simulink model "rippleCarryAdder"  (R2015a)
settings: Solver=ode1  StartTime=0.0  StopTime=10.0  FixedStep=1  RelTol=1e-3
libraries: commutil2 x3
settings Model: Creator=Osmaz  LastModifiedBy=Osmaz

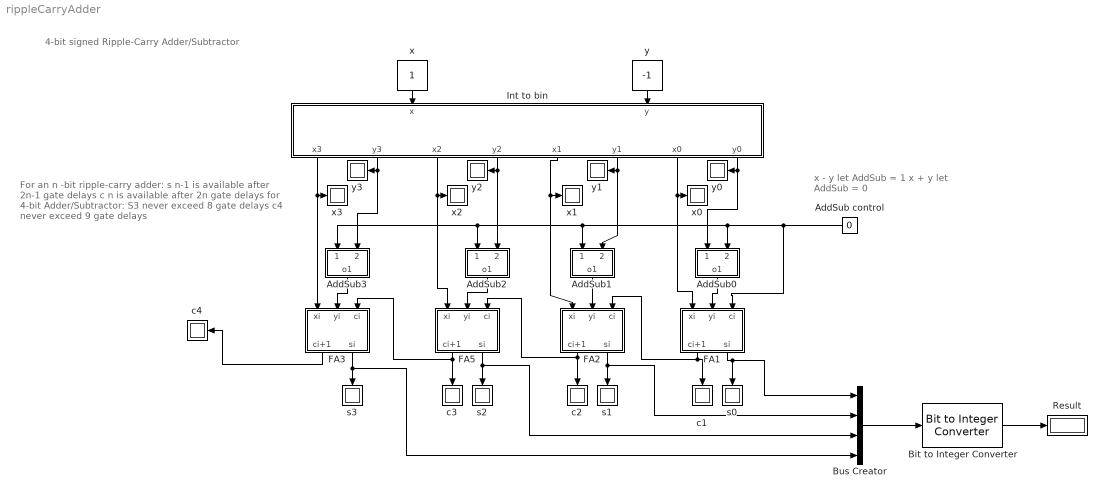
== system rippleCarryAdder ==
  note: For an n -bit ripple-carry adder:
      | s n-1 is available after 2n-1 gate delays
      | c n is available after 2n gate delays
      |
      | for 4-bit Adder/Subtractor:
      | S3 never exceed 8 gate delays
      | c4 never exceed 9 gate delays
  note: 4-bit signed Ripple-Carry Adder/Subtractor
  note: x - y let AddSub = 1
      | x + y let AddSub = 0
  AddSub control : Constant  Value=0  OutMin=0  OutMax=1  OutDataTypeStr=boolean
  AddSub0 : Subsystem
  AddSub1 : Subsystem
  AddSub2 : Subsystem
  AddSub3 : Subsystem
  Bit to Integer Converter : commutil2/Bit to Integer Converter  nbits=4  bitOrder=LSB first  signedOutputValues=Signed  outDtype=Inherit via internal rule  outDtypeSigned=Inherit via internal rule
  Bus Creator : BusCreator  DialogController=Simulink.DDGSource_BusCreator
  FA1 : Subsystem
  FA2 : Subsystem
  FA3 : Subsystem
  FA5 : Subsystem
  Int to bin : Subsystem
  Result : Display
  c{1..4} (4 alike) : Display
  s{0..3} (4 alike) : Display
  x : Constant  OutMin=-8  OutMax=7  OutDataTypeStr=int8  SampleTime=1
  x{0..3} (4 alike) : Display
  y : Constant  Value=-1  OutMin=-8  OutMax=7  OutDataTypeStr=int8  SampleTime=1
  y{0..3} (4 alike) : Display
  wires:
  Int to bin/7(x0) -> x0/1, FA1/1(xi)
  AddSub control/1 -> FA1/3(ci), AddSub1/1(1), AddSub3/1(1), AddSub2/1(1), AddSub0/2(2)
  FA1/2(si) -> s0/1, Bus Creator/1
  Int to bin/5(x1) -> FA2/1(xi), x1/1
  FA2/2(si) -> Bus Creator/2, s1/1
  FA1/1(ci+1) -> c1/1, FA2/3(ci)
  Int to bin/3(x2) -> FA5/1(xi), x2/1
  FA5/2(si) -> s2/1, Bus Creator/3
  FA2/1(ci+1) -> FA5/3(ci), c2/1
  Int to bin/1(x3) -> x3/1, FA3/1(xi)
  FA3/2(si) -> s3/1, Bus Creator/4
  FA5/1(ci+1) -> FA3/3(ci), c3/1
  FA3/1(ci+1) -> c4/1
  Bit to Integer Converter/1 -> Result/1
  Bus Creator/1 -> Bit to Integer Converter/1
  x/1 -> Int to bin/1(x)
  y/1 -> Int to bin/2(y)
  Int to bin/8(y0) -> AddSub0/1(1), y0/1
  Int to bin/6(y1) -> AddSub1/2(2), y1/1
  Int to bin/4(y2) -> y2/1, AddSub2/2(2)
  Int to bin/2(y3) -> AddSub3/2(2), y3/1
  AddSub1/1(o1) -> FA2/2(yi)
  AddSub2/1(o1) -> FA5/2(yi)
  AddSub3/1(o1) -> FA3/2(yi)
  AddSub0/1(o1) -> FA1/2(yi)

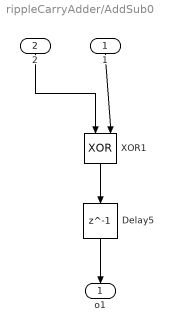
== system rippleCarryAdder/AddSub0 ==
  1 : Inport
  2 : Inport  Port=2
  Delay5 : Delay  DialogController=Simulink.DDGSource  DelayLength=1  InitialCondition=0  InputProcessing=Inherited
  XOR1 : Logic  Operator=XOR  IconShape=distinctive  AllPortsSameDT=off  OutDataTypeStr=boolean
  o1 : Outport
  wires:
  1/1 -> XOR1/2
  2/1 -> XOR1/1
  XOR1/1 -> Delay5/1
  Delay5/1 -> o1/1

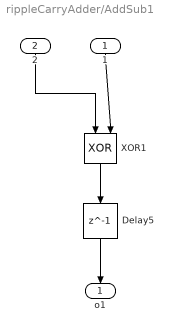
== system rippleCarryAdder/AddSub1 ==
  1 : Inport
  2 : Inport  Port=2
  Delay5 : Delay  DelayLength=1  InitialCondition=0  InputProcessing=Inherited
  XOR1 : Logic  Operator=XOR  IconShape=distinctive  AllPortsSameDT=off  OutDataTypeStr=boolean
  o1 : Outport
  wires:
  1/1 -> XOR1/2
  2/1 -> XOR1/1
  XOR1/1 -> Delay5/1
  Delay5/1 -> o1/1

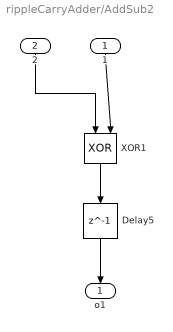
== system rippleCarryAdder/AddSub2 ==
  1 : Inport
  2 : Inport  Port=2
  Delay5 : Delay  DelayLength=1  InitialCondition=0  InputProcessing=Inherited
  XOR1 : Logic  Operator=XOR  IconShape=distinctive  AllPortsSameDT=off  OutDataTypeStr=boolean
  o1 : Outport
  wires:
  1/1 -> XOR1/2
  2/1 -> XOR1/1
  XOR1/1 -> Delay5/1
  Delay5/1 -> o1/1

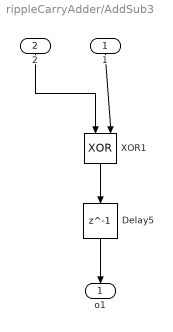
== system rippleCarryAdder/AddSub3 ==
  1 : Inport
  2 : Inport  Port=2
  Delay5 : Delay  DelayLength=1  InitialCondition=0  InputProcessing=Inherited
  XOR1 : Logic  Operator=XOR  IconShape=distinctive  AllPortsSameDT=off  OutDataTypeStr=boolean
  o1 : Outport
  wires:
  1/1 -> XOR1/2
  2/1 -> XOR1/1
  XOR1/1 -> Delay5/1
  Delay5/1 -> o1/1

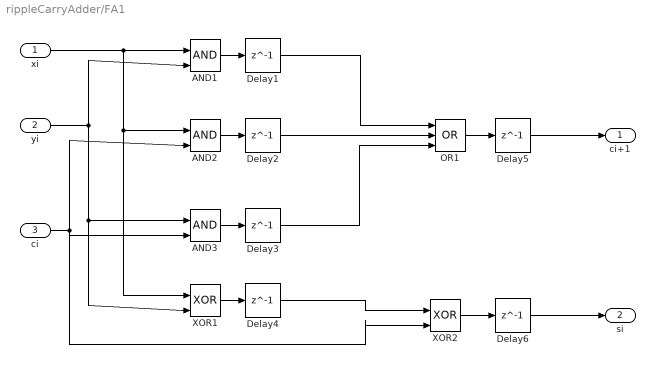
== system rippleCarryAdder/FA1 ==
  xi : Inport
  yi : Inport  Port=2
  ci : Inport  Port=3
  AND1 : Logic  IconShape=distinctive  AllPortsSameDT=off  OutDataTypeStr=boolean
  AND2 : Logic  IconShape=distinctive  AllPortsSameDT=off  OutDataTypeStr=boolean
  AND3 : Logic  IconShape=distinctive  AllPortsSameDT=off  OutDataTypeStr=boolean
  Delay{1..6} (6 alike) : Delay  DelayLength=1  InitialCondition=0  InputProcessing=Inherited
  OR1 : Logic  Operator=OR  Inputs=3  IconShape=distinctive  AllPortsSameDT=off  OutDataTypeStr=boolean
  XOR1 : Logic  Operator=XOR  IconShape=distinctive  AllPortsSameDT=off  OutDataTypeStr=boolean
  XOR2 : Logic  Operator=XOR  IconShape=distinctive  AllPortsSameDT=off  OutDataTypeStr=boolean
  ci+1 : Outport
  si : Outport  Port=2
  wires:
  Delay1/1 -> OR1/1
  AND1/1 -> Delay1/1
  yi/1 -> AND1/2, XOR1/2, AND3/1
  xi/1 -> AND1/1, XOR1/1, AND2/1
  AND2/1 -> Delay2/1
  Delay2/1 -> OR1/2
  AND3/1 -> Delay3/1
  Delay3/1 -> OR1/3
  ci/1 -> XOR2/2, AND2/2, AND3/2
  OR1/1 -> Delay5/1
  Delay5/1 -> ci+1/1
  Delay6/1 -> si/1
  XOR1/1 -> Delay4/1
  Delay4/1 -> XOR2/1
  XOR2/1 -> Delay6/1

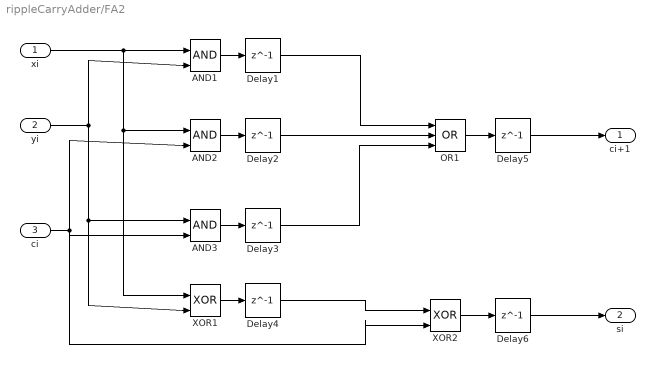
== system rippleCarryAdder/FA2 ==
  xi : Inport
  yi : Inport  Port=2
  ci : Inport  Port=3
  AND1 : Logic  IconShape=distinctive  AllPortsSameDT=off  OutDataTypeStr=boolean
  AND2 : Logic  IconShape=distinctive  AllPortsSameDT=off  OutDataTypeStr=boolean
  AND3 : Logic  IconShape=distinctive  AllPortsSameDT=off  OutDataTypeStr=boolean
  Delay{1..6} (6 alike) : Delay  DelayLength=1  InitialCondition=0  InputProcessing=Inherited
  OR1 : Logic  Operator=OR  Inputs=3  IconShape=distinctive  AllPortsSameDT=off  OutDataTypeStr=boolean
  XOR1 : Logic  Operator=XOR  IconShape=distinctive  AllPortsSameDT=off  OutDataTypeStr=boolean
  XOR2 : Logic  Operator=XOR  IconShape=distinctive  AllPortsSameDT=off  OutDataTypeStr=boolean
  ci+1 : Outport
  si : Outport  Port=2
  wires:
  Delay1/1 -> OR1/1
  AND1/1 -> Delay1/1
  yi/1 -> AND1/2, XOR1/2, AND3/1
  xi/1 -> AND1/1, XOR1/1, AND2/1
  AND2/1 -> Delay2/1
  Delay2/1 -> OR1/2
  AND3/1 -> Delay3/1
  Delay3/1 -> OR1/3
  ci/1 -> XOR2/2, AND2/2, AND3/2
  OR1/1 -> Delay5/1
  Delay5/1 -> ci+1/1
  Delay6/1 -> si/1
  XOR1/1 -> Delay4/1
  Delay4/1 -> XOR2/1
  XOR2/1 -> Delay6/1

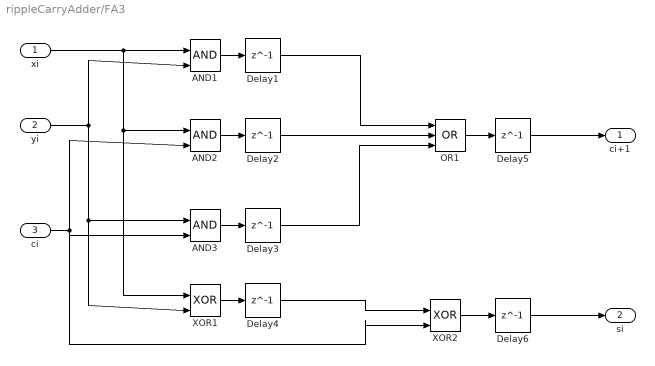
== system rippleCarryAdder/FA3 ==
  xi : Inport
  yi : Inport  Port=2
  ci : Inport  Port=3
  AND1 : Logic  IconShape=distinctive  AllPortsSameDT=off  OutDataTypeStr=boolean
  AND2 : Logic  IconShape=distinctive  AllPortsSameDT=off  OutDataTypeStr=boolean
  AND3 : Logic  IconShape=distinctive  AllPortsSameDT=off  OutDataTypeStr=boolean
  Delay{1..6} (6 alike) : Delay  DelayLength=1  InitialCondition=0  InputProcessing=Inherited
  OR1 : Logic  Operator=OR  Inputs=3  IconShape=distinctive  AllPortsSameDT=off  OutDataTypeStr=boolean
  XOR1 : Logic  Operator=XOR  IconShape=distinctive  AllPortsSameDT=off  OutDataTypeStr=boolean
  XOR2 : Logic  Operator=XOR  IconShape=distinctive  AllPortsSameDT=off  OutDataTypeStr=boolean
  ci+1 : Outport
  si : Outport  Port=2
  wires:
  Delay1/1 -> OR1/1
  AND1/1 -> Delay1/1
  yi/1 -> AND1/2, XOR1/2, AND3/1
  xi/1 -> AND1/1, XOR1/1, AND2/1
  AND2/1 -> Delay2/1
  Delay2/1 -> OR1/2
  AND3/1 -> Delay3/1
  Delay3/1 -> OR1/3
  ci/1 -> XOR2/2, AND2/2, AND3/2
  OR1/1 -> Delay5/1
  Delay5/1 -> ci+1/1
  Delay6/1 -> si/1
  XOR1/1 -> Delay4/1
  Delay4/1 -> XOR2/1
  XOR2/1 -> Delay6/1

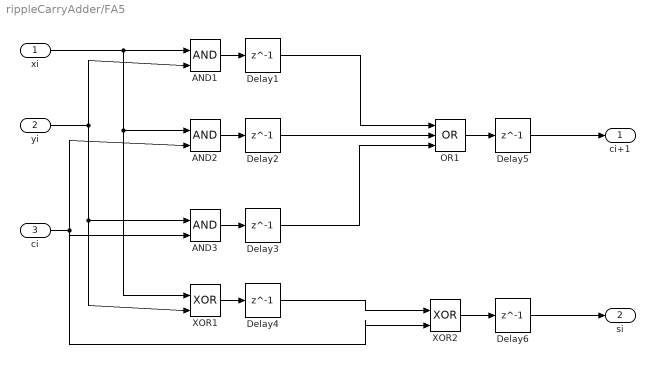
== system rippleCarryAdder/FA5 ==
  xi : Inport
  yi : Inport  Port=2
  ci : Inport  Port=3
  AND1 : Logic  IconShape=distinctive  AllPortsSameDT=off  OutDataTypeStr=boolean
  AND2 : Logic  IconShape=distinctive  AllPortsSameDT=off  OutDataTypeStr=boolean
  AND3 : Logic  IconShape=distinctive  AllPortsSameDT=off  OutDataTypeStr=boolean
  Delay{1..6} (6 alike) : Delay  DelayLength=1  InitialCondition=0  InputProcessing=Inherited
  OR1 : Logic  Operator=OR  Inputs=3  IconShape=distinctive  AllPortsSameDT=off  OutDataTypeStr=boolean
  XOR1 : Logic  Operator=XOR  IconShape=distinctive  AllPortsSameDT=off  OutDataTypeStr=boolean
  XOR2 : Logic  Operator=XOR  IconShape=distinctive  AllPortsSameDT=off  OutDataTypeStr=boolean
  ci+1 : Outport
  si : Outport  Port=2
  wires:
  Delay1/1 -> OR1/1
  AND1/1 -> Delay1/1
  yi/1 -> AND1/2, XOR1/2, AND3/1
  xi/1 -> AND1/1, XOR1/1, AND2/1
  AND2/1 -> Delay2/1
  Delay2/1 -> OR1/2
  AND3/1 -> Delay3/1
  Delay3/1 -> OR1/3
  ci/1 -> XOR2/2, AND2/2, AND3/2
  OR1/1 -> Delay5/1
  Delay5/1 -> ci+1/1
  Delay6/1 -> si/1
  XOR1/1 -> Delay4/1
  Delay4/1 -> XOR2/1
  XOR2/1 -> Delay6/1

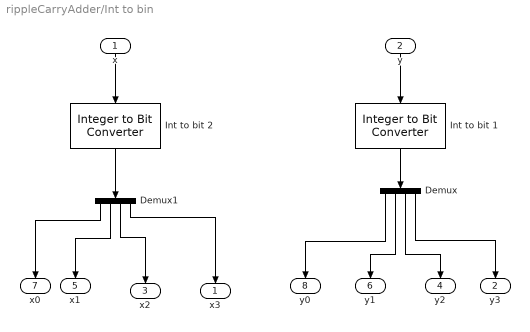
== system rippleCarryAdder/Int to bin ==
  x : Inport
  y : Inport  Port=2
  Demux : Demux
  Demux1 : Demux
  Int to bit 1 : commutil2/Integer to Bit Converter  nbits=4  signedInputValues=Signed  bitOrder=LSB first  outDtype=Inherit via internal rule
  Int to bit 2 : commutil2/Integer to Bit Converter  nbits=4  signedInputValues=Signed  bitOrder=LSB first  outDtype=Inherit via internal rule
  x3 : Outport
  y3 : Outport  Port=2
  x2 : Outport  Port=3
  y2 : Outport  Port=4
  x1 : Outport  Port=5
  y1 : Outport  Port=6
  x0 : Outport  Port=7
  y0 : Outport  Port=8
  wires:
  Demux1/1 -> x0/1
  Demux/2 -> y1/1
  Demux1/2 -> x1/1
  Demux/1 -> y0/1
  y/1 -> Int to bit 1/1
  Int to bit 1/1 -> Demux/1
  x/1 -> Int to bit 2/1
  Demux1/3 -> x2/1
  Demux1/4 -> x3/1
  Demux/3 -> y2/1
  Int to bit 2/1 -> Demux1/1
  Demux/4 -> y3/1
